simulink library "VideoProcessingLib"  (R2016a)
settings: Solver=ode45  StartTime=0.0  StopTime=10.0  RelTol=1e-3
libraries: GreenBallTracking x1
settings Model: Creator=sannem  LastModifiedBy=sannem
settings DataIOCC: LimitDataPoints=on
settings DebuggingCC: AllowSymbolicDim=off

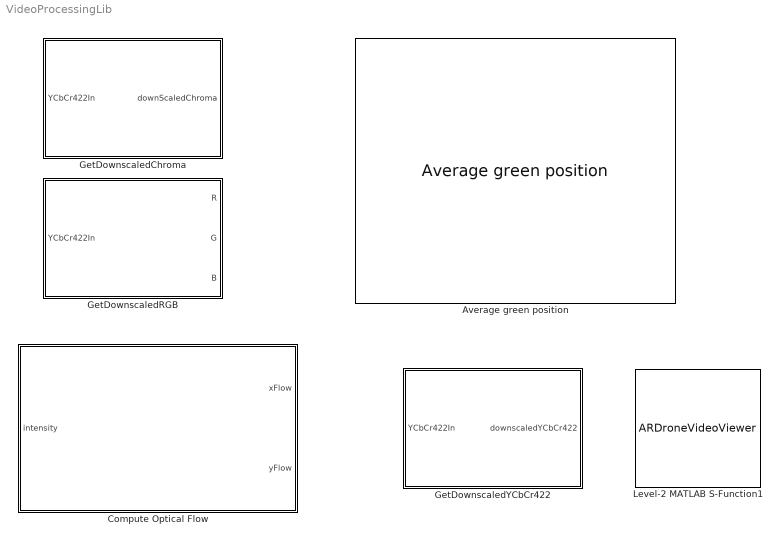
== system VideoProcessingLib ==
  Average green position : GreenBallTracking/Average green position  width=1280  height=720  downScaleFactor=4
  "Compute Optical Flow " : MATLAB Function  TreatAsAtomicUnit=on  mask(Optical flow){bufferSize=8}
      mask prompts: bufferSize "Frame buffer size"
      mask help: This block takes a matrix of intensity values and computes the X and Y flow componenets from the difference between the user specified number of frames (minimum of 3). Increasing the frame buffer reduces noise but increases latency.
  "GetDownscaledChroma " : MATLAB Function  TreatAsAtomicUnit=on  mask(Down scaled chromatic){width=320, height=240, downScaleFactor=8}
      mask prompts: width "Input Image width"; height "Input Image height"; downScaleFactor "Down scaling factor"
      mask help: This Block downscales the chromatic value of a YCrCb input stream and outputs it as a matrix of intensity values
  "GetDownscaledRGB " : MATLAB Function  TreatAsAtomicUnit=on  mask(Down scaled chromatic){width=1280, height=720, downScaleFactor=8}
      mask prompts: width "Input Image width"; height "Input Image height"; downScaleFactor "Down scaling factor"
      mask help: This Block downscales the chromatic value of a YCrCb input stream and outputs it as a matrix of intensity values
  GetDownscaledYCbCr422 : MATLAB Function  TreatAsAtomicUnit=on  mask(Down scaled chromatic){width=1280, height=720, downScaleFactor=8}
      mask prompts: width "Input Image width"; height "Input Image height"; downScaleFactor "Down scaling factor"
      mask help: This Block downscales the chromatic value of a YCrCb input stream and outputs it as a matrix of intensity values
  Level-2 MATLAB S-Function1 : M-S-Function  FunctionName=ARDroneVideoViewer  Parameters=horAspect,verAspect  mask{horAspect=16, verAspect=9}
      mask prompts: horAspect "Horizontal video aspect ratio"; verAspect "Vertical video aspect ratio"

== matlab function VideoProcessingLib/GetDownscaledRGB  ==
  data: YCbCr422In input; R output; width parameter; height parameter; downScaleFactor parameter; G output; B output

function [R,G,B]   = GetDownscaledRGB(YCbCr422In,width, height, downScaleFactor)
 
R = uint8(zeros(height/downScaleFactor,width/2/downScaleFactor));
G = uint8(zeros(height/downScaleFactor,width/2/downScaleFactor));
B = uint8(zeros(height/downScaleFactor,width/2/downScaleFactor));
if ~isempty(YCbCr422In)

    %% constants for color conversion
    c1 =     298.082/256;
    Rc1 =    408.583/256;
    Rc2 =   -222.921;
    Gc1 =   -100.291/256;
    Gc2 =   -208.120/256;
    Gc3 =    135.576;
    Bc1=     516.412/256;
    Bc2=    -276.836;

    %% Downsample and convert to RGB

    for verticalIndex = 1 : 1 : height/downScaleFactor;             % indexing for downsampled vertical direction
        for horizontalIndex = 1 : 1 : (width / 2)/downScaleFactor;  % indexing for downsampled horizontal direction
            index = 4 * (downScaleFactor * (verticalIndex - 1) * (width / 2) + downScaleFactor * horizontalIndex) - 3;  % translate the horizontal and vertical indexes into the index into the video input
            pixel = [single(YCbCr422In(index)) single(YCbCr422In(index+1)) single(YCbCr422In(index+2)) single(YCbCr422In(index+3))];
            yFactor = c1 * (pixel(2)+pixel(4))/2;  % Average the chroma value
            R(verticalIndex, horizontalIndex) = yFactor + Rc1 * pixel(3) + Rc2;
            G(verticalIndex, horizontalIndex) = yFactor + Gc1 * pixel(1) + Gc2 * pixel(3) + Gc3;
            B(verticalIndex, horizontalIndex) = yFactor + Bc1 * pixel(1) + Rc2;
        end
    end
end
end

== matlab function VideoProcessingLib/GetDownscaledYCbCr422 ==
  data: YCbCr422In input; downscaledYCbCr422 output; width parameter; height parameter; downScaleFactor parameter

function downscaledYCbCr422    = GetDownscaledYCbCr4S22(YCbCr422In, width, height, downScaleFactor)

%% Downsample and convert to RGB

outputLength = width * height * 2 / downScaleFactor / downScaleFactor;
downscaledYCbCr422 = uint8( zeros( outputLength, 1) );

outputIndex = 1;
for verticalIndex = 1 : 1 : height/downScaleFactor;             % indexing for downsampled vertical direction
    for horizontalIndex = 1 : 1 : (width / 2)/downScaleFactor;  % indexing for downsampled horizontal direction
        index = 4 * (downScaleFactor * (verticalIndex - 1) * (width / 2) + downScaleFactor * horizontalIndex) - 3;  % translate the horizontal and vertical indexes into the index into the video input
        downscaledYCbCr422(outputIndex : outputIndex + 3) = uint8(YCbCr422In(index : index + 3));
        outputIndex = outputIndex + 4;
    end
end
end

== matlab function VideoProcessingLib/GetDownscaledChroma  ==
  data: YCbCr422In input; downScaledChroma output; width parameter; height parameter; downScaleFactor parameter

function downScaledChroma   = GetDownscaledChroma(YCbCr422In,width, height, downScaleFactor)

downScaledChroma = uint8(zeros(height/downScaleFactor,width/downScaleFactor));

for verticalIndex = 1 : 1 : height/downScaleFactor;             % indexing for downsampled vertical direction
    for horizontalIndex = 1 : 1 : (width / 2)/downScaleFactor;  % indexing for downsampled horizontal direction
        index = 4 * (downScaleFactor * (verticalIndex - 1) * (width / 2) + downScaleFactor * horizontalIndex) - 3;  % translate the horizontal and vertical indexes into the index into the video input
        downScaledChroma(verticalIndex, 2 * horizontalIndex - 1) = YCbCr422In(index + 1);
        downScaledChroma(verticalIndex, 2 * horizontalIndex) = YCbCr422In(index+3);
    end
end
end

== matlab function VideoProcessingLib/Compute Optical Flow  ==
  data: intensity input; xFlow output; yFlow output; bufferSize parameter
function [xFlow,yFlow]   = ComputeOpticalFlow(intensity,bufferSize)

persistent maxDiffs maxVals imageBuffer;




if isempty(maxDiffs)
    maxDiffs = zeros(2,bufferSize - 1);
else
    maxDiffs (:,2:end) = maxDiffs(:,1:end - 1);
    maxDiffs (:,1) = [0;0];
end

if isempty(maxVals)
    maxVals = zeros(2,bufferSize - 1);
else
    maxVals (:,2:end) = maxVals(:,1:end - 1);
    maxVals (:,1) = [0;0];
end

if isempty(imageBuffer) %initialize
   imageBuffer = intensity;
end


[width,height] = size(intensity);

xFlow = 0;
yFlow = 0;

bufferDifference = abs( int16(intensity) - int16(imageBuffer) );
[maxVals(1,1),maxDiffs(1,1)] = max( max( bufferDifference, [], 1) ); 
[maxVals(2,1),maxDiffs(2,1)] = max( max( bufferDifference, [], 2) ); 

xMax = sum(maxVals(1,:))
yMax = sum(maxVals(2,:))

for k = 1 : bufferSize - 2;
    xFlow = xFlow + maxDiffs(1,k) - maxDiffs(1,k+1);
    yFlow = yFlow + maxDiffs(2,k) - maxDiffs(2,k+1);
end

imageBuffer = intensity;   %save the current frame for next itteration

xFlow = xFlow / (bufferSize - 2) * xMax / (bufferSize - 1) / 100; 
yFlow = yFlow / (bufferSize - 2) * yMax / (bufferSize - 1) / 100;
end
